simulink model "q_aero_free_osc_response_pitch"  (R2014a)
settings: Solver=ode1  StartTime=0.0  StopTime=30  FixedStep=0.002  RelTol=1e-3
libraries: quarc_library x2, quanser_aero x1
settings Model: SimulationMode=external  ExtModeTrigDuration=15000  Creator=MLevis  LastModifiedBy=MLevis
settings SolverCC: PositivePriorityOrder=on
settings DebuggingCC: MergeDetectMultiDrivingBlocksExec=error
settings RTWCC: SystemTargetFile=quarc_win64.tlc  TemplateMakefile=quarc_default_tmf  Description=QUARC Win64 Target  ProcessScript=quarc_win64_make_rtw_hook
settings GRTTargetCC: ParMdlRefBuildCompliant=off  CompOptLevelCompliant=off  CombineOutputUpdateFcns=off  MatFileLogging=off  CPPClassGenCompliant=off  GRTInterface=on  ExtMode=on  ExtModeMexFile=quarc_comm

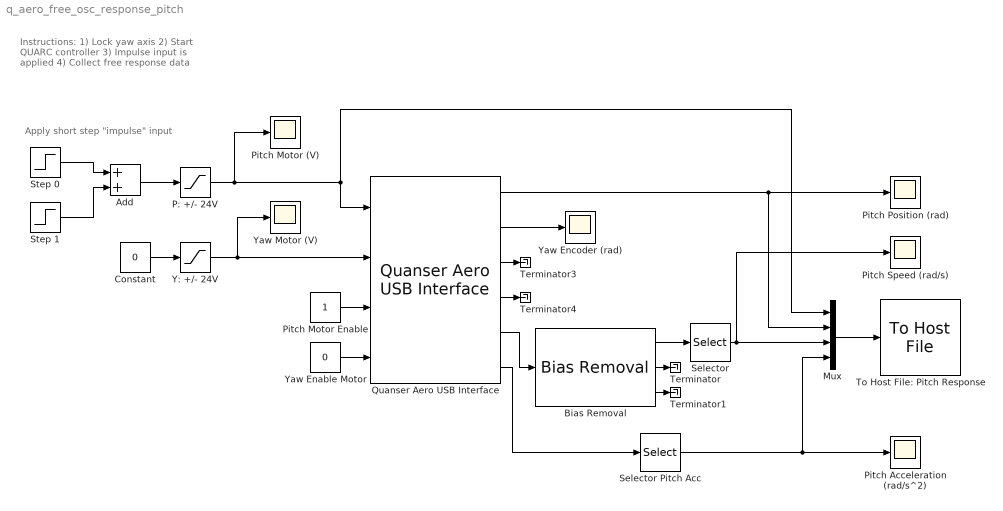
== system q_aero_free_osc_response_pitch ==
  note: Apply short step "impulse" input
  note: Instructions:
      | 1) Lock yaw axis
      | 2) Start QUARC controller
      | 3) Impulse input is applied
      | 4) Collect free response data
  Add : Sum
  Bias Removal : quarc_library/Discrete/Bias Removal  start_time=0  end_time=1  switch_id=0  sample_time=qc_get_step_size
  Constant : Constant  Value=0
  Mux : Mux
  P: +/- 24V : Saturate  UpperLimit=24  LowerLimit=-24
  Pitch Acceleration (rad/s^2) : Scope
      settings: TimeRange=30  YMin=-10  YMax=10  SaveName=pitch_spd1  MaxDataPoints=15000
  Pitch Motor (V) : Scope
      settings: TimeRange=30  YMin=-25  YMax=25  SaveName=ScopeData2  MaxDataPoints=15000
  Pitch Motor Enable : Constant
  Pitch Position (rad) : Scope
      settings: TimeRange=30  YMin=-1.5  YMax=1.5  SaveName=ScopeData3  MaxDataPoints=15000
  Pitch Speed (rad/s) : Scope
      settings: TimeRange=30  YMin=-1.5  YMax=1.5  SaveName=pitch_spd  MaxDataPoints=15000
  Quanser Aero USB Interface : quanser_aero/Quanser Aero USB Interface
  Selector : Selector  InputPortWidth=3  Indices=[2]
  Selector Pitch Acc : Selector  InputPortWidth=3  Indices=[1]
  Step 0 : Step  After=-20  SampleTime=0
  Step 1 : Step  Time=1.75  After=20  SampleTime=0
  Terminator{,1,3..4} (4 alike) : Terminator
  To Host File: Pitch Response : quarc_library/Sinks/To Host/To Host File  file_name=aero_pitch_free_osc_rsp.mat  variable_name=free_osc_rsp_pitch  decimation=1  sample_time=-1  file_format=MAT-file v.4  options=No header or footer  append=off  final_file_name=aero_pitch_free_osc_rsp.mat
  Y: +/- 24V : Saturate  UpperLimit=24  LowerLimit=-24
  Yaw Enable Motor : Constant  Value=0
  Yaw Encoder (rad) : Scope
      settings: TimeRange=5  YMin=-0.5  YMax=1.5  SaveName=ScopeData4
  Yaw Motor (V) : Scope
      settings: TimeRange=5  YMin=-25  YMax=25  SaveName=ScopeData5
  wires:
  Pitch Motor Enable/1 -> Quanser Aero USB Interface/3
  Yaw Enable Motor/1 -> Quanser Aero USB Interface/4
  Y: +/- 24V/1 -> Quanser Aero USB Interface/2, Yaw Motor (V)/1
  P: +/- 24V/1 -> Quanser Aero USB Interface/1, Mux/1, Pitch Motor (V)/1
  Quanser Aero USB Interface/1 -> Mux/2, Pitch Position (rad)/1
  Quanser Aero USB Interface/2 -> Yaw Encoder (rad)/1
  Mux/1 -> To Host File: Pitch Response/1
  Bias Removal/2 -> Terminator/1
  Bias Removal/3 -> Terminator1/1
  Quanser Aero USB Interface/3 -> Terminator3/1
  Quanser Aero USB Interface/4 -> Terminator4/1
  Bias Removal/1 -> Selector/1
  Selector/1 -> Mux/3, Pitch Speed (rad/s)/1
  Selector Pitch Acc/1 -> Pitch Acceleration (rad/s^2)/1, Mux/4
  Quanser Aero USB Interface/5 -> Bias Removal/1
  Quanser Aero USB Interface/6 -> Selector Pitch Acc/1
  Constant/1 -> Y: +/- 24V/1
  Step 0/1 -> Add/1
  Step 1/1 -> Add/2
  Add/1 -> P: +/- 24V/1
